simulink subsystem "CollectivePitchControl"  (R2022a)
settings: Solver=VariableStepAuto  StartTime=0.0  StopTime=10.0  RelTol=1e-3
undefined symbols (not defined in the file): F, R, simu
libraries: simulink x1
settings Model: Creator=jhummel  LastModifiedBy=jhummel

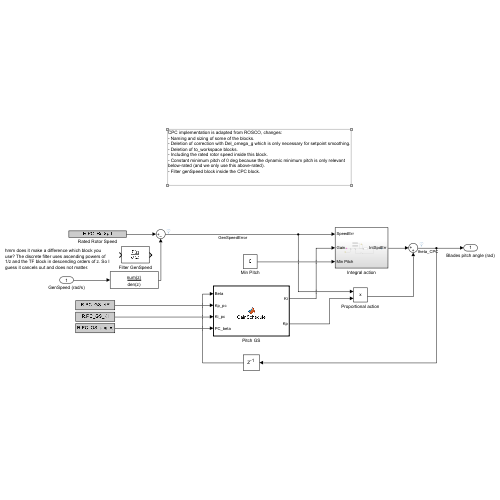
[thumbnail: Simulink's stored preview of the top-level diagram]
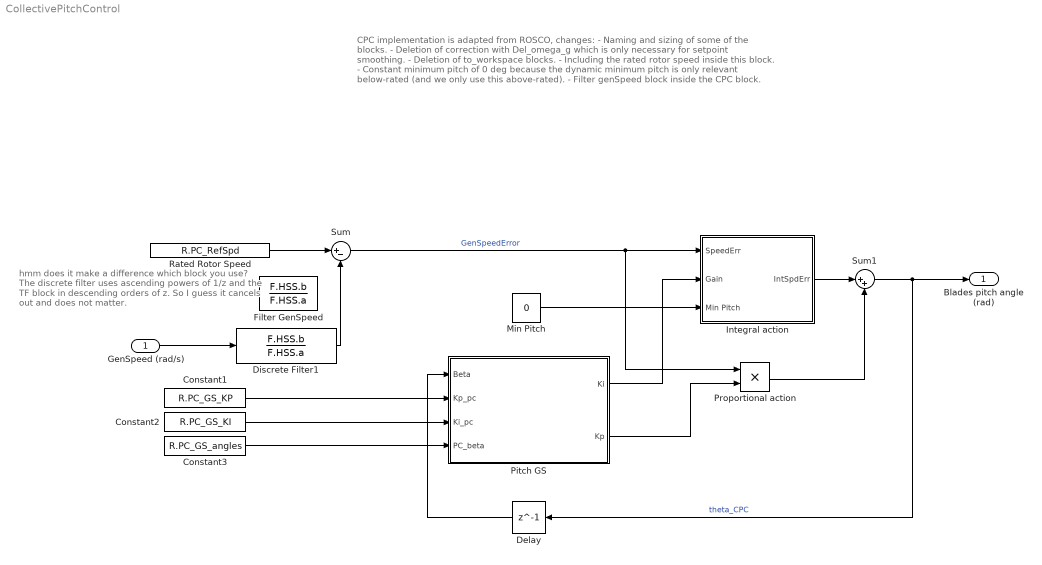
== system CollectivePitchControl ==
  note: hmm does it make a difference which block you use? The discrete filter uses ascending powers of 1/z and the TF block in descending orders of z. So I guess it cancels out and does not matter.
  note: CPC implementation is adapted from ROSCO, changes:
      | - Naming and sizing of some of the blocks.
      | - Deletion of correction with Del_omega_g which is only necessary for setpoint smoothing.
      | - Deletion of to_workspace blocks.
      | - Including the rated rotor speed inside this block.
      | - Constant minimum pitch of 0 deg because the dynamic minimum pitch is only relevant below-rated (and we only use this above-rated).
      | - Filter genSpeed block inside the CPC block.
  GenSpeed (rad/s) : Inport
  Constant1 : Constant  Value=R.PC_GS_KP
  Constant2 : Constant  Value=R.PC_GS_KI
  Constant3 : Constant  Value=R.PC_GS_angles
  Delay : Delay  DelayLength=1
  Discrete Filter1 : DiscreteFilter  Numerator=F.HSS.b  Denominator=F.HSS.a  InitialStates=R.VS_RefSpd/(sum(F.HSS.a(2:end))+1)
  Filter GenSpeed : DiscreteTransferFcn  Numerator=F.HSS.b  Denominator=F.HSS.a  InitialStates=R.VS_RefSpd/(sum(F.HSS.a(2:end))+1)
  Integral action : Subsystem
  Min Pitch : Constant  Value=0
  Pitch GS : MATLAB Function  TreatAsAtomicUnit=on
  Proportional action : Product
  Rated Rotor Speed : Constant  Value=R.PC_RefSpd
  Sum : Sum  Inputs=|+-
  Sum1 : Sum  Inputs=|++
  Blades pitch angle (rad) : Outport
  wires:
  Delay/1 -> Pitch GS/1(Beta)
  Constant3/1 -> Pitch GS/4(PC_beta)
  Integral action/1(IntSpdErr) -> Sum1/1
  Constant1/1 -> Pitch GS/2(Kp_pc)
  Sum1/1 -> Delay/1, Blades pitch angle (rad)/1  "theta_CPC"
  Proportional action/1 -> Sum1/2
  Pitch GS/1(Ki) -> Integral action/2(Gain)
  Pitch GS/2(Kp) -> Proportional action/2
  Constant2/1 -> Pitch GS/3(Ki_pc)
  GenSpeed (rad/s)/1 -> Discrete Filter1/1
  Sum/1 -> Integral action/1(SpeedErr), Proportional action/1  "GenSpeedError"
  Rated Rotor Speed/1 -> Sum/1
  Min Pitch/1 -> Integral action/3(Min Pitch)
  Discrete Filter1/1 -> Sum/2

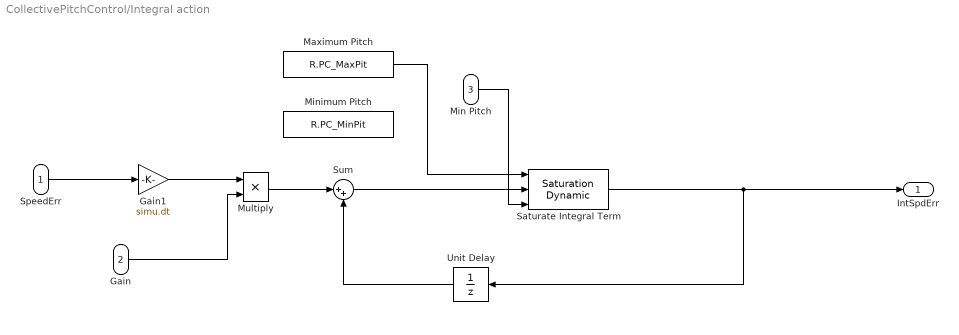
== system CollectivePitchControl/Integral action ==
  SpeedErr : Inport
  Gain : Inport  Port=2
  Min Pitch : Inport  Port=3
  Gain1 : Gain  Gain=simu.dt
  Maximum Pitch : Constant  Value=R.PC_MaxPit
  Minimum Pitch : Constant  Value=R.PC_MinPit
  Multiply : Product
  Saturate Integral Term : simulink/Discontinuities/Saturation Dynamic  OutMin=[]  OutMax=[]  OutDataTypeStr=Inherit: Same as second input  OutDataType=fixdt(1, 16)  OutScaling=2^-10  RndMeth=Nearest  DoSatur=off
  Sum : Sum  Inputs=|++
  Unit Delay : UnitDelay  InitialCondition=deg2rad(11)  SampleTime=-1  HasFrameUpgradeWarning=on
  IntSpdErr : Outport  VectorParamsAs1DForOutWhenUnconnected=off
  wires:
  Min Pitch/1 -> Saturate Integral Term/3
  Multiply/1 -> Sum/1
  Gain1/1 -> Multiply/1
  Saturate Integral Term/1 -> Unit Delay/1, IntSpdErr/1
  Gain/1 -> Multiply/2
  SpeedErr/1 -> Gain1/1
  Sum/1 -> Saturate Integral Term/2
  Unit Delay/1 -> Sum/2
  Maximum Pitch/1 -> Saturate Integral Term/1

== matlab function CollectivePitchControl/Pitch GS ==
  data: Ki output size=1; Beta input; Kp_pc input; Kp output size=1; Ki_pc input; PC_beta input
function [Ki, Kp] = GainSchedule(Beta, Kp_pc, Ki_pc,  PC_beta)

% This function calculates the current gains for a Collective Blade Pitch 
% controller
%
% Inputs: v - Current wind speed estimate, m/s.
%         ContParam - Structure of control parameters, output from
%                     ControlParameters.m
%
% Outputs: Kp - Proportional Gain
%          Ki - Integral Gain
%
% Nikhar Abbas - May 2019


%% Linear Gain Schedule
% pKp_pc = ContParam.GS.pKp_pc;
% pKi_pc = ContParam.GS.pKi_pc;
% 
% %%
% Kp = pKp_pc(1)*Beta + pKp_pc(2);
% Ki = pKi_pc(1)*Beta + pKi_pc(2);
% % Kp = pKp_pc(1)*v + pKp_pc(2)
% % Ki = pKi_pc(1)*v + pKi_pc(2);
% 
% Kpmax = pKp_pc(1)*15*pi/180 + pKp_pc(2);
% Kimax = pKi_pc(1)*15*pi/180 + pKi_pc(2);
% 
% Kp = min(Kp, Kpmax);
% Ki = min(Ki,Kimax);

%% nonlinear Gain Schedule
% Kp_pc   = R.PC_GS_KP;
% Ki_pc   = R.PC_GS_KI;
% PC_beta = R.PC_GS_angles;

beta    = max(min(Beta,PC_beta(end)), PC_beta(1));

% gains
Kp      = interp1(PC_beta,Kp_pc, beta);
Ki      = interp1(PC_beta,Ki_pc, beta);



end
